simulink model "LinearTopObserver"  (R2019a)
settings: Solver=VariableStepAuto  StartTime=0.0  StopTime=10  RelTol=1e-3
values from neighbouring files (symbols this model uses):
  Parameters = CoenParams(X)    [EstimatedParams.m]    (also in LQR.m = EstimatedParams(); LSQnonLinfunc.m; TestModel.m = CoenParams(X0); testingLQRDisturbance.m = EstimatedParams())
settings Model: Creator=coeng  LastModifiedBy=coeng
settings DebuggingCC: ArithmeticOperatorsInVariantConditions=warning
settings CodeAppCC: StateflowObjectComments=on

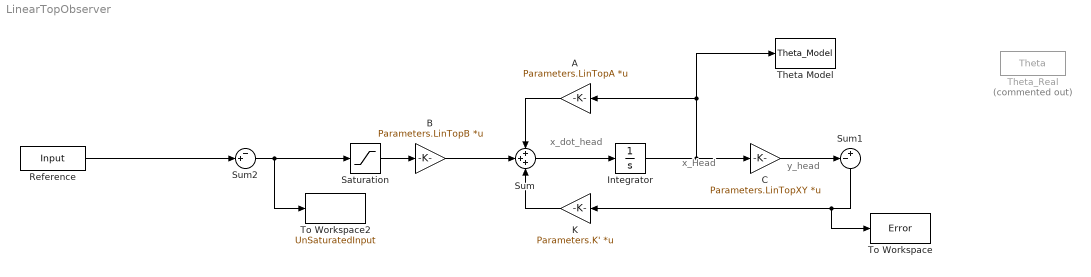
== system LinearTopObserver ==
  note: y_head
  note: x_dot_head
  note: x_Head
  A : Gain  Gain=Parameters.LinTopA  Multiplication=Matrix(K*u)
  B : Gain  Gain=Parameters.LinTopB  Multiplication=Matrix(K*u)
  C : Gain  Gain=Parameters.LinTopXY  Multiplication=Matrix(K*u)
  Integrator : Integrator
  K : Gain  Gain=Parameters.K'  Multiplication=Matrix(K*u)
  "Reference " : FromWorkspace  VariableName=Input  SampleTime=0
  Saturation : Saturate  UpperLimit=1  LowerLimit=-1
  Sum : Sum  Inputs=+++
  Sum1 : Sum  Inputs=-+|
  Sum2 : Sum  Inputs=-+|
  Theta Model : ToWorkspace  VariableName=Theta_Model  SaveFormat=Timeseries  SampleTime=-1
  Theta_Real : FromWorkspace  Commented=on  VariableName=Theta  SampleTime=0
  To Workspace : ToWorkspace  VariableName=Error  SaveFormat=Timeseries  SampleTime=-1
  To Workspace2 : ToWorkspace  VariableName=UnSaturatedInput  SaveFormat=Timeseries  SampleTime=-1
  wires:
  Sum/1 -> Integrator/1
  Integrator/1 -> C/1, A/1, Theta Model/1
  Sum2/1 -> To Workspace2/1, Saturation/1
  Saturation/1 -> B/1
  Sum1/1 -> K/1, To Workspace/1
  K/1 -> Sum/3
  C/1 -> Sum1/1
  A/1 -> Sum/1
  B/1 -> Sum/2
  "Reference "/1 -> Sum2/2
